simulink library "qt_opengl_visualization_lib"  (R2018b)
settings: Solver=VariableStepAuto  StartTime=0.0  StopTime=10.0  RelTol=1e-3
undefined symbols (not defined in the file or in its folder): aircraft, aircraft_double_array, aircraft_double_idx
libraries: dspnetwork x1
settings Model: Creator=yannic  LastModifiedBy=yannic

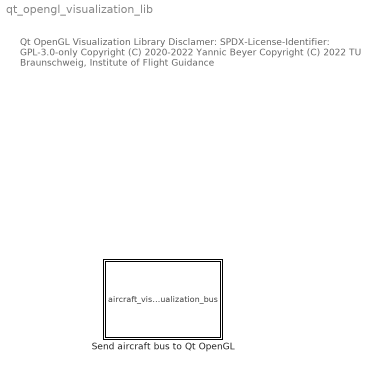
== system qt_opengl_visualization_lib ==
  note: Qt OpenGL Visualization Library
      |
      | Disclamer:
      | SPDX-License-Identifier: GPL-3.0-only
      |
      | Copyright (C) 2020-2022 Yannic Beyer
      | Copyright (C) 2022 TU Braunschweig, Institute of Flight Guidance
  Send aircraft bus to Qt OpenGL : Subsystem  mask{sample_time=1/30, ip_address='192.168.11.13', ip_port=4321, aircraft=aircraft}
      mask prompts: sample_time "sample time"; ip_address "IP address"; ip_port "IP port"; aircraft "aircraft parameters struct"
      mask init:
      | [aircraft_visualization,aircraft_double_array,aircraft_double_idx] ...
      |     = aircraftCreateVisualizer(aircraft);
      | [aircraft_double_array,aircraft_double_idx] = struct2double(aircraft_visualization,999999);

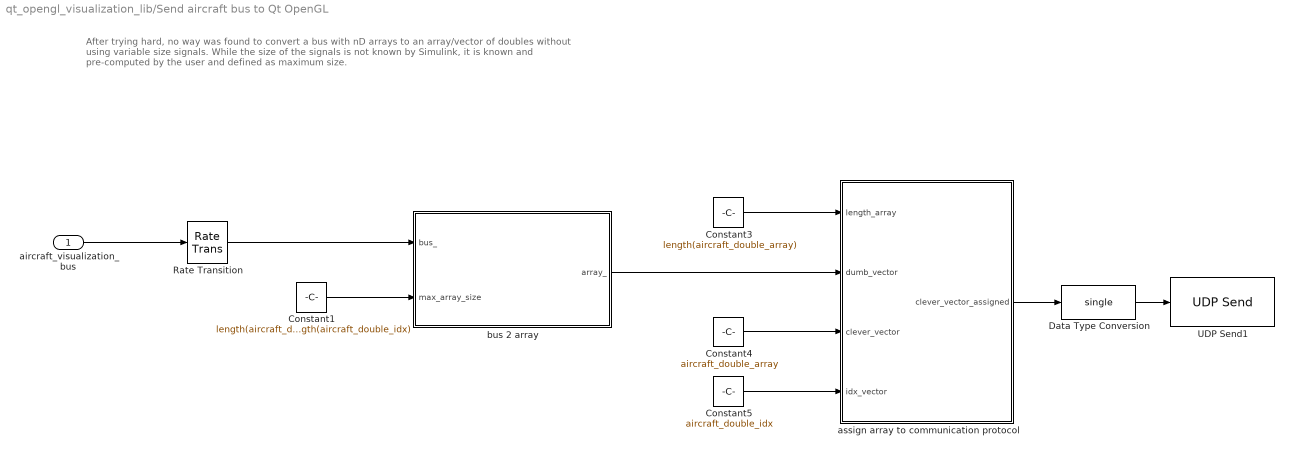
== system qt_opengl_visualization_lib/Send aircraft bus to Qt OpenGL ==
  note: After trying hard, no way was found to convert a bus with nD arrays to an array/vector of doubles without using variable size signals.
      | While the size of the signals is not known by Simulink, it is known and pre-computed by the user and defined as maximum size.
  aircraft_visualization_bus : Inport
  Constant1 : Constant  Value=length(aircraft_double_array)-length(aircraft_double_idx)
  Constant3 : Constant  Value=length(aircraft_double_array)
  Constant4 : Constant  Value=aircraft_double_array
  Constant5 : Constant  Value=aircraft_double_idx
  Data Type Conversion : DataTypeConversion  OutDataTypeStr=single
  Rate Transition : RateTransition  OutPortSampleTime=sample_time
  UDP Send1 : dspnetwork/UDP Send  remoteURL=ip_address  remotePort=ip_port  localURL='0.0.0.0'  localPortSource=Automatically determine  localPort=-1  sampletime=-1  blockPlatform=[]  separateLengthPort=0
      settings: SourceProductName=Simulink
  assign array to communication protocol : MATLAB Function  TreatAsAtomicUnit=on
  bus 2 array : MATLAB Function  TreatAsAtomicUnit=on
  wires:
  Data Type Conversion/1 -> UDP Send1/1
  bus 2 array/1(array_) -> assign array to communication protocol/2(dumb_vector)
  Constant5/1 -> assign array to communication protocol/4(idx_vector)
  Constant4/1 -> assign array to communication protocol/3(clever_vector)
  Constant3/1 -> assign array to communication protocol/1(length_array)
  assign array to communication protocol/1(clever_vector_assigned) -> Data Type Conversion/1
  Rate Transition/1 -> bus 2 array/1(bus_)
  aircraft_visualization_bus/1 -> Rate Transition/1
  Constant1/1 -> bus 2 array/2(max_array_size)

== matlab function qt_opengl_visualization_lib/Send aircraft bus to Qt OpenGL/bus 2 array ==
  data: bus_ input; array_ output size=[1, length(aircraft_double_array)-length(aircraft_double_idx)]; max_array_size input
function array_ = fcn(bus_,max_array_size)

array_ = bus2array(bus_,max_array_size);

== matlab function qt_opengl_visualization_lib/Send aircraft bus to Qt OpenGL/assign array to communication protocol ==
  data: length_array input; dumb_vector input size=[1, length(aircraft_double_array)-length(aircraft_double_idx)]; clever_vector input; idx_vector input; clever_vector_assigned output size=[1, length(aircraft_double_array)+1]
function clever_vector_assigned = fcn(length_array, dumb_vector,clever_vector, idx_vector)

clever_vector_row = clever_vector(:)';
idx_vector_row = idx_vector(:)';

clever_out = clever_vector_row;

clever_out(idx_vector_row) = clever_vector_row(idx_vector_row);
% inverse index
idx_2 = setdiff(1:length(clever_out),idx_vector_row);
clever_out(idx_2) = dumb_vector(1:length(idx_2));
clever_vector_assigned = [ length_array, clever_out ];
